simulink library "Lib_DQTrans_dqs2dqe"  (R2021a)
settings: Solver=VariableStepAuto  StartTime=0.0  StopTime=10.0  RelTol=1e-3
settings Model: Creator=30610  LastModifiedBy=30610

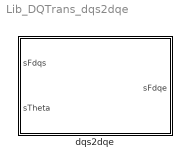
== system Lib_DQTrans_dqs2dqe ==
  dqs2dqe : Subsystem

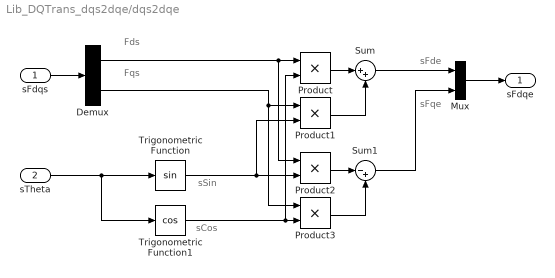
== system Lib_DQTrans_dqs2dqe/dqs2dqe ==
  note: sFqe
  note: sFde
  note: sCos
  note: sSin
  note: Fqs
  note: Fds
  sFdqs : Inport
  sTheta : Inport  Port=2
  Demux : Demux  Outputs=2
  Mux : Mux  Inputs=2
  Product{,1..3} (4 alike) : Product  RndMeth=Zero
  Sum : Sum  Inputs=|++
  Sum1 : Sum  Inputs=|-+
  Trigonometric Function : Trigonometry
  Trigonometric Function1 : Trigonometry  Operator=cos
  sFdqe : Outport  VectorParamsAs1DForOutWhenUnconnected=off
  wires:
  Product/1 -> Sum/1
  Product3/1 -> Sum1/2
  Demux/1 -> Product2/1, Product/1
  Trigonometric Function1/1 -> Product/2, Product3/2
  sFdqs/1 -> Demux/1
  Trigonometric Function/1 -> Product1/2, Product2/2
  Product1/1 -> Sum/2
  Demux/2 -> Product3/1, Product1/1
  Product2/1 -> Sum1/1
  Mux/1 -> sFdqe/1
  Sum/1 -> Mux/1
  Sum1/1 -> Mux/2
  sTheta/1 -> Trigonometric Function1/1, Trigonometric Function/1
